simulink model "tut06b"  (R2025a)
settings: Solver=VariableStepAuto  StartTime=0.0  StopTime=10.0  RelTol=1e-3
libraries: NSA_DEVS_LOGISTICS x5, NSA_DEVS_SINKS x4, NSA_DEVS_ROUTING x2, NSA_DEVS_SOURCES x1
settings Model: Creator=peter  LastModifiedBy=peter

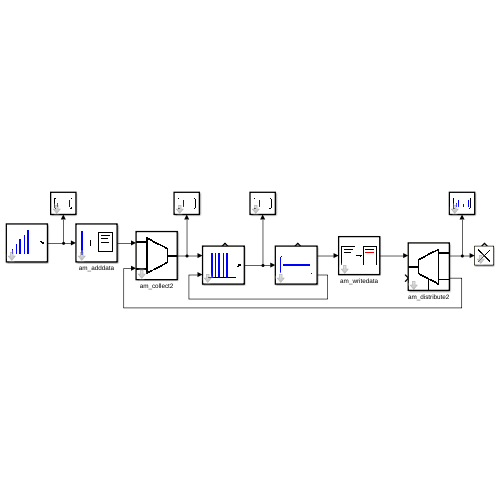
[thumbnail: Simulink's stored preview of the top-level diagram]
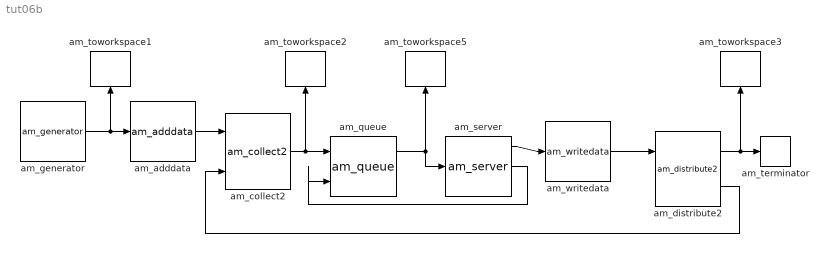
== system tut06b ==
  am_adddata : NSA_DEVS_LOGISTICS/am_adddata  fields="[\"outPort\"]"  values="[\"0\"]"  numeric=[true]  infield="\"id\""  tau=[0,1]  debug=0
      settings: SourceProductName=Logistics
  am_collect2 : NSA_DEVS_ROUTING/am_collect2  tD=[0,2]  tau=[0,1]  debug=0
      settings: SourceProductName=Routing
  am_distribute2 : NSA_DEVS_ROUTING/am_distribute2  port0=1  field="\"outPort\""  tau=[0,1]  debug=0
      settings: SourceProductName=Routing
  am_generator : NSA_DEVS_SOURCES/am_generator  tG=1  n0=1  nG=6  tD=[0,2]  debug=0
      settings: SourceProductName=Sources
  am_queue : NSA_DEVS_LOGISTICS/am_queue  tD=[0,2]  tau=[0,1]  debug=0
      settings: SourceProductName=Logistics
  am_server : NSA_DEVS_LOGISTICS/am_server  tS=1  tsField="\"\""  tau=[0,1]  debug=0
      settings: SourceProductName=Logistics
  am_terminator : NSA_DEVS_LOGISTICS/am_terminator  tau=[0,1]  debug=0
      settings: SourceProductName=Logistics
  am_toworkspace1 : NSA_DEVS_SINKS/am_toworkspace  varname="\"gen\""  t0=0  format="\"vector\""  tau=[0,5]  debug=0
      settings: SourceProductName=Sinks
  am_toworkspace2 : NSA_DEVS_SINKS/am_toworkspace  varname="\"qIn\""  t0=0  format="\"vector\""  tau=[0,0.5]  debug=0
      settings: SourceProductName=Sinks
  am_toworkspace3 : NSA_DEVS_SINKS/am_toworkspace  varname="\"sysOut\""  t0=0  format="\"vector\""  tau=[0,5]  debug=0
      settings: SourceProductName=Sinks
  am_toworkspace5 : NSA_DEVS_SINKS/am_toworkspace  varname="\"qOut\""  t0=0  format="\"vector\""  tau=[0,5]  debug=0
      settings: SourceProductName=Sinks
  am_writedata : NSA_DEVS_LOGISTICS/am_writedata  inFields=[]  outField="\"outPort\""  changeFunc="\"out = (rand() > 0.5) + 1;\""  tau=[0,1]  debug=0
      settings: SourceProductName=Logistics
  wires:
  am_collect2/1 -> am_queue/1, am_toworkspace2/1
  am_queue/1 -> am_toworkspace5/1, am_server/1
  am_server/2 -> am_queue/2
  am_generator/1 -> am_toworkspace1/1, am_adddata/1
  am_adddata/1 -> am_collect2/1
  am_server/1 -> am_writedata/1
  am_writedata/1 -> am_distribute2/1
  am_distribute2/1 -> am_toworkspace3/1, am_terminator/1
  am_distribute2/2 -> am_collect2/2
